simulink model "AE623_Burder_MakeupQuiz2_Problem2_LKF_EKF"  (R2016b)
settings: Solver=VariableStepAuto  StartTime=0.0  StopTime=10800  RelTol=1e-3
values from neighbouring files (symbols this model uses):
  T = 0.1    [AE623_Burder_MakeupQuiz2_Problem1.m]    (also in UKF.m = times)
undefined symbols (not defined in the file or in its folder): DiscIntNeverNeededParam
settings Model: Creator=burderd  LastModifiedBy=burderd

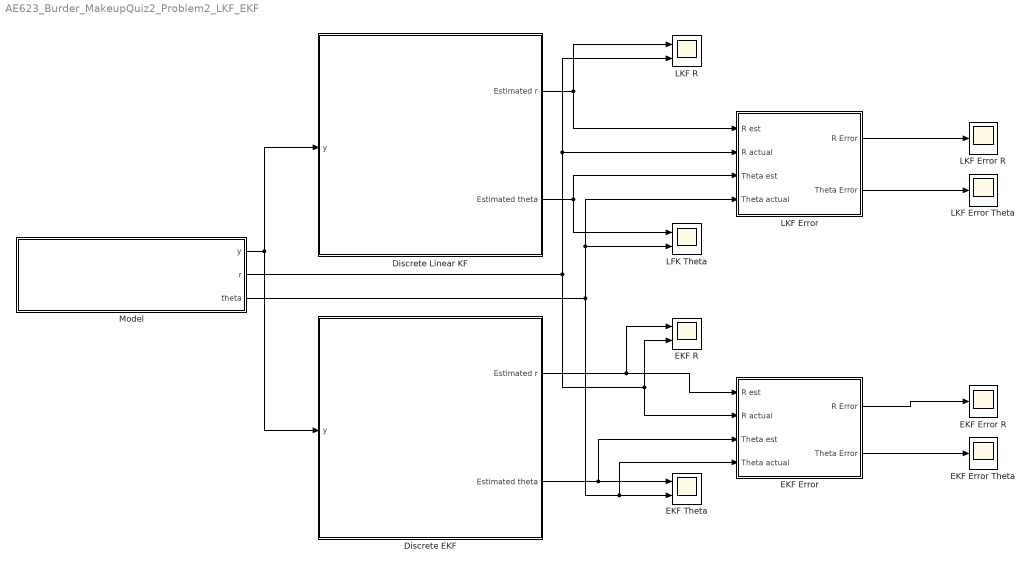
== system AE623_Burder_MakeupQuiz2_Problem2_LKF_EKF ==
  " EKF Error Theta" : Scope
  " EKF Theta" : Scope  NumInputPorts=2
  " LFK Theta" : Scope  NumInputPorts=2
  " LKF Error Theta" : Scope
  Discrete EKF : Subsystem  mask{Td=1, G=6.66742e-11, M=5.98e24, w0=0.011171034854823, r0=1.57e6}
  Discrete Linear KF : Subsystem  mask{Td=1, G=6.66742e-11, M=5.98e24, w0=0.011171034854823, r0=1.57e6}
  EKF Error : Subsystem
  EKF Error R : Scope
  EKF R : Scope  NumInputPorts=2
  LKF Error : Subsystem
  LKF Error R : Scope
  LKF R : Scope  NumInputPorts=2
  Model : Subsystem
  wires:
  Model/1(y) -> Discrete Linear KF/1(y), Discrete EKF/1(y)
  Discrete Linear KF/1(Estimated r) -> LKF R/1, LKF Error/1(R est)
  Discrete Linear KF/2(Estimated theta) -> LKF Error/3(Theta est), " LFK Theta"/1
  Model/2(r) -> EKF Error/2(R actual), EKF R/2, LKF R/2, LKF Error/2(R actual)
  Model/3(theta) -> " LFK Theta"/2, LKF Error/4(Theta actual), EKF Error/4(Theta actual), " EKF Theta"/2
  Discrete EKF/1(Estimated r) -> EKF Error/1(R est), EKF R/1
  Discrete EKF/2(Estimated theta) -> EKF Error/3(Theta est), " EKF Theta"/1
  LKF Error/1(R Error) -> LKF Error R/1
  LKF Error/2(Theta Error) -> " LKF Error Theta"/1
  EKF Error/1(R Error) -> EKF Error R/1
  EKF Error/2(Theta Error) -> " EKF Error Theta"/1

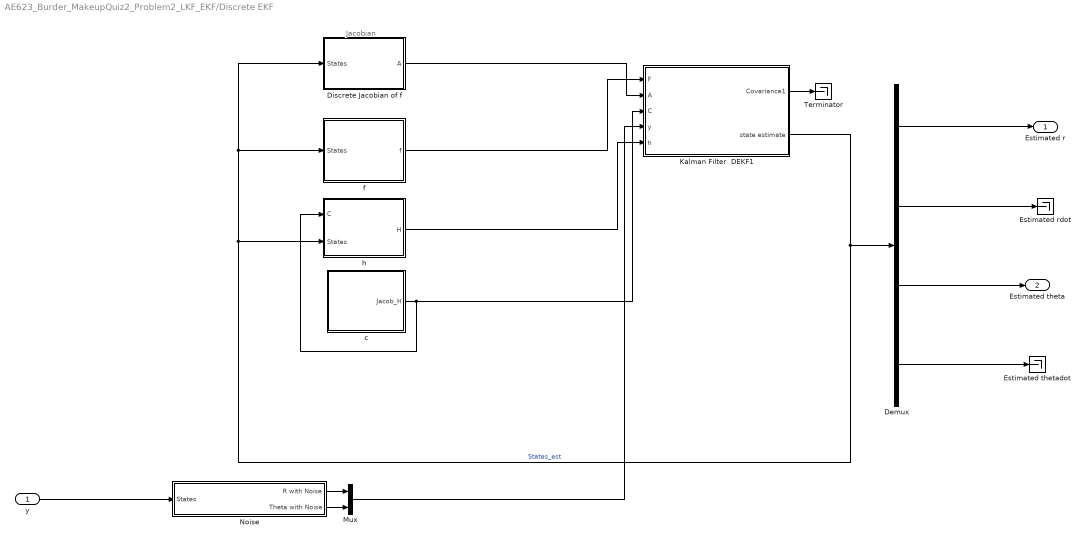
== system AE623_Burder_MakeupQuiz2_Problem2_LKF_EKF/Discrete EKF ==
  note: Jacobian
  y : Inport
  Demux : Demux
  Discrete Jacobian of f : Subsystem
  Estimated rdot : Terminator
  Estimated thetadot : Terminator
  Kalman Filter  DEKF1 : Subsystem
  Mux : Mux  Inputs=2
  Noise : Subsystem
  Terminator : Terminator
  c : Subsystem
  "f " : Subsystem
  h : Subsystem
  Estimated r : Outport
  Estimated theta : Outport  Port=2
  wires:
  Mux/1 -> Kalman Filter  DEKF1/4(y)
  y/1 -> Noise/1(States)
  Noise/2(Theta with Noise) -> Mux/2
  Noise/1(R with Noise) -> Mux/1
  h/1(H) -> Kalman Filter  DEKF1/5(h)
  Kalman Filter  DEKF1/2(state estimate) -> Demux/1, h/2(States), Discrete Jacobian of f/1(States), "f "/1(States)  "States_est"
  Kalman Filter  DEKF1/1(Covariance1) -> Terminator/1
  c/1(Jacob_H) -> h/1(C), Kalman Filter  DEKF1/3(C)
  "f "/1(f) -> Kalman Filter  DEKF1/1(F)
  Demux/1 -> Estimated r/1
  Demux/2 -> Estimated rdot/1
  Demux/3 -> Estimated theta/1
  Demux/4 -> Estimated thetadot/1
  Discrete Jacobian of f/1(A) -> Kalman Filter  DEKF1/2(A)

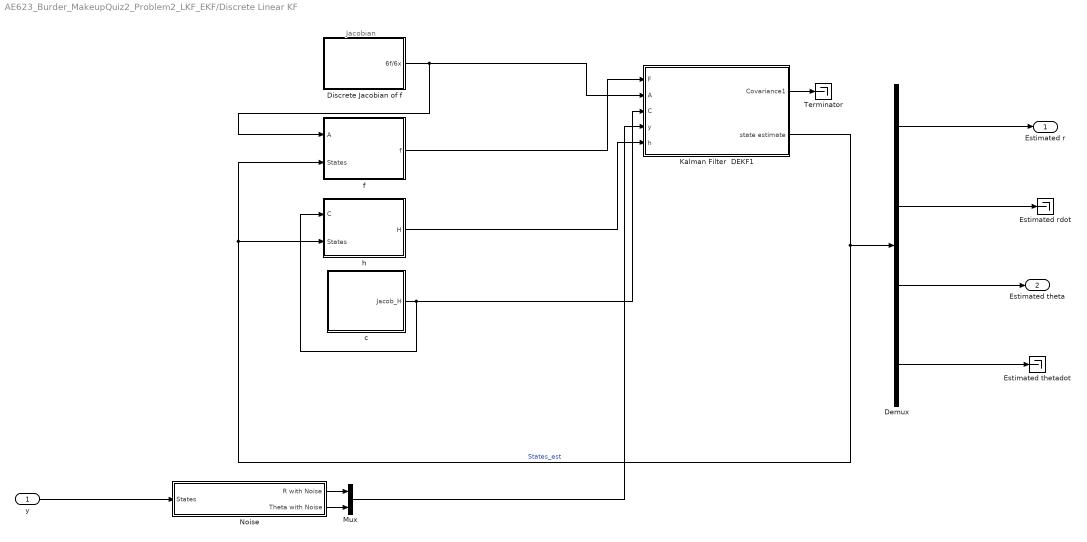
== system AE623_Burder_MakeupQuiz2_Problem2_LKF_EKF/Discrete Linear KF ==
  note: Jacobian
  y : Inport
  Demux : Demux
  Discrete Jacobian of f : Subsystem
  Estimated rdot : Terminator
  Estimated thetadot : Terminator
  Kalman Filter  DEKF1 : Subsystem
  Mux : Mux  Inputs=2
  Noise : Subsystem
  Terminator : Terminator
  c : Subsystem
  "f " : Subsystem
  h : Subsystem
  Estimated r : Outport
  Estimated theta : Outport  Port=2
  wires:
  Demux/4 -> Estimated thetadot/1
  Demux/3 -> Estimated theta/1
  Demux/2 -> Estimated rdot/1
  Demux/1 -> Estimated r/1
  Discrete Jacobian of f/1(6f/6x) -> Kalman Filter  DEKF1/2(A), "f "/1(A)
  "f "/1(f) -> Kalman Filter  DEKF1/1(F)
  c/1(Jacob_H) -> Kalman Filter  DEKF1/3(C), h/1(C)
  Kalman Filter  DEKF1/1(Covariance1) -> Terminator/1
  Kalman Filter  DEKF1/2(state estimate) -> "f "/2(States), h/2(States), Demux/1  "States_est"
  h/1(H) -> Kalman Filter  DEKF1/5(h)
  Noise/1(R with Noise) -> Mux/1
  Noise/2(Theta with Noise) -> Mux/2
  y/1 -> Noise/1(States)
  Mux/1 -> Kalman Filter  DEKF1/4(y)

== system AE623_Burder_MakeupQuiz2_Problem2_LKF_EKF/EKF Error ==
  R est : Inport
  R actual : Inport  Port=2
  Theta est : Inport  Port=3
  Theta actual : Inport  Port=4
  Sum2 : Sum  Inputs=|+-
  Sum3 : Sum  Inputs=|+-
  R Error : Outport
  Theta Error : Outport  Port=2
  wires:
  Theta est/1 -> Sum3/2
  R actual/1 -> Sum2/1
  R est/1 -> Sum2/2
  Theta actual/1 -> Sum3/1
  Sum2/1 -> R Error/1
  Sum3/1 -> Theta Error/1

== system AE623_Burder_MakeupQuiz2_Problem2_LKF_EKF/LKF Error ==
  R est : Inport
  R actual : Inport  Port=2
  Theta est : Inport  Port=3
  Theta actual : Inport  Port=4
  Sum2 : Sum  Inputs=|+-
  Sum3 : Sum  Inputs=|+-
  R Error : Outport
  Theta Error : Outport  Port=2
  wires:
  Theta est/1 -> Sum3/2
  R actual/1 -> Sum2/1
  R est/1 -> Sum2/2
  Theta actual/1 -> Sum3/1
  Sum2/1 -> R Error/1
  Sum3/1 -> Theta Error/1

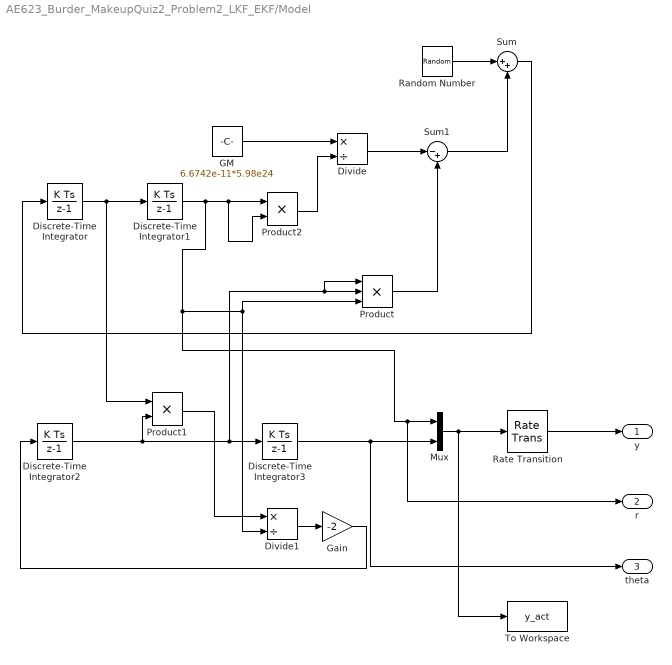
== system AE623_Burder_MakeupQuiz2_Problem2_LKF_EKF/Model ==
  Discrete-Time Integrator : DiscreteIntegrator  InitialConditionSetting=State (most efficient)  SampleTime=-1  ICPrevOutput=DiscIntNeverNeededParam  ICPrevScaledInput=DiscIntNeverNeededParam
  Discrete-Time Integrator1 : DiscreteIntegrator  InitialCondition=1.57e6  InitialConditionSetting=State (most efficient)  SampleTime=-1  ICPrevOutput=DiscIntNeverNeededParam  ICPrevScaledInput=DiscIntNeverNeededParam
  Discrete-Time Integrator2 : DiscreteIntegrator  InitialCondition=1.1*sqrt(6.6742e-11*5.98e24/(1.57e6)^3)  InitialConditionSetting=State (most efficient)  SampleTime=-1  ICPrevOutput=DiscIntNeverNeededParam  ICPrevScaledInput=DiscIntNeverNeededParam
  Discrete-Time Integrator3 : DiscreteIntegrator  InitialConditionSetting=State (most efficient)  SampleTime=-1  ICPrevOutput=DiscIntNeverNeededParam  ICPrevScaledInput=DiscIntNeverNeededParam
  Divide : Product  Inputs=*/
  Divide1 : Product  Inputs=*/
  GM : Constant  Value=6.6742e-11*5.98e24
  Gain : Gain  Gain=-2
  Mux : Mux  Inputs=2
  Product : Product  Inputs=3
  Product1 : Product
  Product2 : Product
  Random Number : RandomNumber  Variance=10e-6
  Rate Transition : RateTransition  X0=[1.57e6 0]  OutPortSampleTime=60
  Sum : Sum  Inputs=|++
  Sum1 : Sum  Inputs=|-+
  To Workspace : ToWorkspace  VariableName=y_act  SaveFormat=Timeseries  SampleTime=-1
  y : Outport
  r : Outport  Port=2
  theta : Outport  Port=3
  wires:
  Divide/1 -> Sum1/1
  Random Number/1 -> Sum/1
  GM/1 -> Divide/1
  Sum/1 -> Discrete-Time Integrator/1
  Sum1/1 -> Sum/2
  Discrete-Time Integrator/1 -> Product1/1, Discrete-Time Integrator1/1
  Discrete-Time Integrator3/1 -> theta/1, Mux/2
  Discrete-Time Integrator1/1 -> Product2/2, Product2/1, Divide1/2, Product/3, r/1, Mux/1
  Discrete-Time Integrator2/1 -> Product1/2, Product/1, Product/2, Discrete-Time Integrator3/1
  Mux/1 -> To Workspace/1, Rate Transition/1
  Product1/1 -> Divide1/1
  Divide1/1 -> Gain/1
  Product/1 -> Sum1/2
  Gain/1 -> Discrete-Time Integrator2/1
  Product2/1 -> Divide/2
  Rate Transition/1 -> y/1

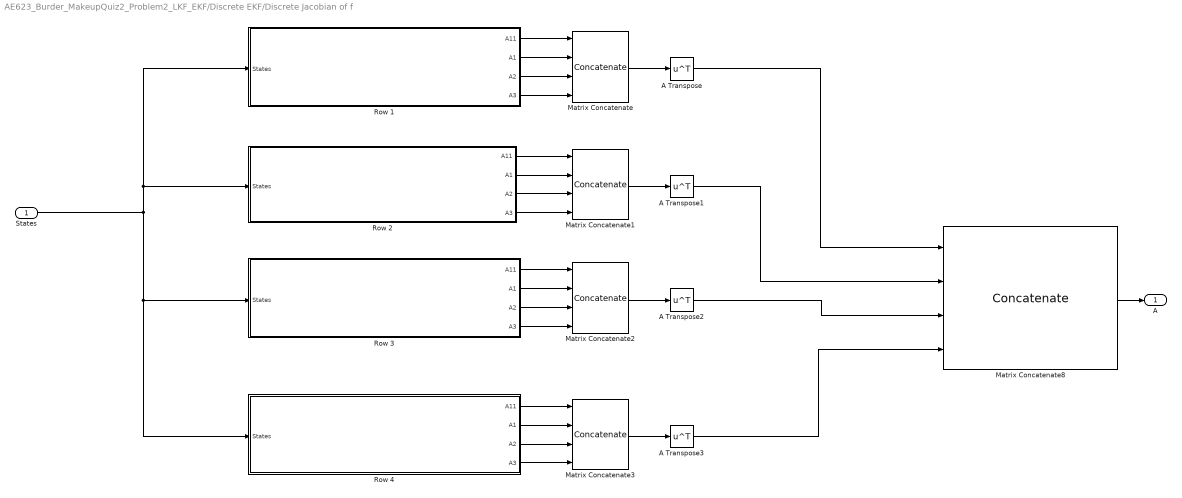
== system AE623_Burder_MakeupQuiz2_Problem2_LKF_EKF/Discrete EKF/Discrete Jacobian of f ==
  States : Inport
  A Transpose{,1..3} (4 alike) : Math  Operator=transpose  SaturateOnIntegerOverflow=on
  Matrix Concatenate{,1..3} (4 alike) : Concatenate  NumInputs=4  ConcatenateDimension=2
  Matrix Concatenate8 : Concatenate  NumInputs=4  Mode=Multidimensional array
  Row 1 : Subsystem
  Row 2 : Subsystem
  Row 3 : Subsystem
  Row 4 : Subsystem
  A : Outport
  wires:
  Matrix Concatenate8/1 -> A/1
  Row 1/1(A11) -> Matrix Concatenate/1
  Row 1/2(A1) -> Matrix Concatenate/2
  Row 1/3(A2) -> Matrix Concatenate/3
  Row 1/4(A3) -> Matrix Concatenate/4
  Matrix Concatenate/1 -> A Transpose/1
  A Transpose/1 -> Matrix Concatenate8/1
  Row 2/1(A11) -> Matrix Concatenate1/1
  Row 2/2(A1) -> Matrix Concatenate1/2
  Row 2/3(A2) -> Matrix Concatenate1/3
  Row 2/4(A3) -> Matrix Concatenate1/4
  Matrix Concatenate1/1 -> A Transpose1/1
  Row 3/1(A11) -> Matrix Concatenate2/1
  Row 3/2(A1) -> Matrix Concatenate2/2
  Row 3/3(A2) -> Matrix Concatenate2/3
  Row 3/4(A3) -> Matrix Concatenate2/4
  Matrix Concatenate2/1 -> A Transpose2/1
  Row 4/1(A11) -> Matrix Concatenate3/1
  Row 4/2(A1) -> Matrix Concatenate3/2
  Row 4/3(A2) -> Matrix Concatenate3/3
  Row 4/4(A3) -> Matrix Concatenate3/4
  Matrix Concatenate3/1 -> A Transpose3/1
  A Transpose1/1 -> Matrix Concatenate8/2
  A Transpose2/1 -> Matrix Concatenate8/3
  A Transpose3/1 -> Matrix Concatenate8/4
  States/1 -> Row 2/1(States), Row 1/1(States), Row 3/1(States), Row 4/1(States)

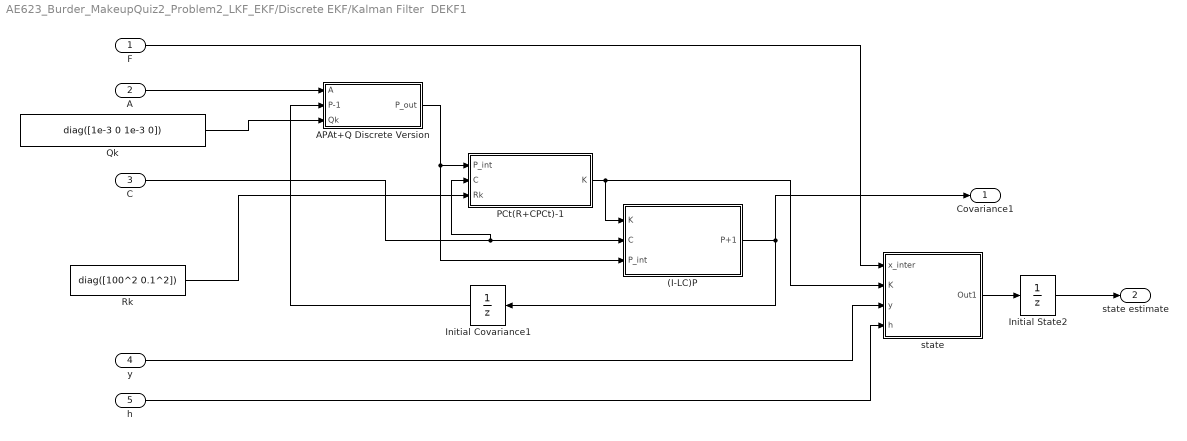
== system AE623_Burder_MakeupQuiz2_Problem2_LKF_EKF/Discrete EKF/Kalman Filter  DEKF1 ==
  F : Inport
  A : Inport  Port=2
  C : Inport  Port=3
  y : Inport  Port=4
  h : Inport  Port=5
  (I-LC)P : Subsystem
  APAt+Q Discrete Version : Subsystem
  Initial Covariance1 : UnitDelay  InitialCondition=zeros(4,4)  SampleTime=Td
  Initial State2 : UnitDelay  InitialCondition=[1.57e6 0 0 1.1*w0]  SampleTime=Td
  PCt(R+CPCt)-1 : Subsystem
  Qk : Constant  Value=diag([1e-3 0 1e-3 0])
  Rk : Constant  Value=diag([100^2 0.1^2])
  state : Subsystem
  Covariance1 : Outport
  state estimate : Outport  Port=2
  wires:
  F/1 -> state/1(x_inter)
  Initial State2/1 -> state estimate/1
  state/1(Out1) -> Initial State2/1
  Initial Covariance1/1 -> APAt+Q Discrete Version/2(P-1)
  PCt(R+CPCt)-1/1(K) -> (I-LC)P/1(K), state/2(K)
  (I-LC)P/1(P+1) -> Initial Covariance1/1, Covariance1/1
  Qk/1 -> APAt+Q Discrete Version/3(Qk)
  APAt+Q Discrete Version/1(P_out) -> (I-LC)P/3(P_int), PCt(R+CPCt)-1/1(P_int)
  A/1 -> APAt+Q Discrete Version/1(A)
  C/1 -> PCt(R+CPCt)-1/2(C), (I-LC)P/2(C)
  y/1 -> state/3(y)
  h/1 -> state/4(h)
  Rk/1 -> PCt(R+CPCt)-1/3(Rk)

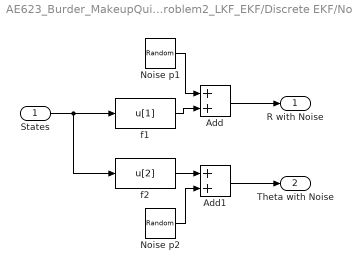
== system AE623_Burder_MakeupQuiz2_Problem2_LKF_EKF/Discrete EKF/Noise ==
  States : Inport
  Add : Sum
  Add1 : Sum
  Noise p1 : RandomNumber  Variance=100  Seed=565  SampleTime=T
  Noise p2 : RandomNumber  Variance=0.1  Seed=525  SampleTime=T
  f1 : Fcn  Expr=u[1]
  f2 : Fcn  Expr=u[2]
  R with Noise : Outport
  Theta with Noise : Outport  Port=2
  wires:
  f2/1 -> Add1/1
  Noise p2/1 -> Add1/2
  Add1/1 -> Theta with Noise/1
  States/1 -> f1/1, f2/1
  f1/1 -> Add/2
  Noise p1/1 -> Add/1
  Add/1 -> R with Noise/1

== system AE623_Burder_MakeupQuiz2_Problem2_LKF_EKF/Discrete EKF/c ==
  note: u[1] =p
      | u[2]=q
      | u[3]=r
      | u[4]=bank_est
      | u[5]=pitch_est
      | u[6]=heading_est
  Matrix Concatenate11 : Concatenate  Mode=Multidimensional array
  Row 1 : Subsystem
  Row 2 : Subsystem
  Jacob_H : Outport
  wires:
  Row 1/1(A11) -> Matrix Concatenate11/1
  Matrix Concatenate11/1 -> Jacob_H/1
  Row 2/1(A21) -> Matrix Concatenate11/2

== system AE623_Burder_MakeupQuiz2_Problem2_LKF_EKF/Discrete EKF/f  ==
  States : Inport
  Matrix Concatenate8 : Concatenate  NumInputs=4  Mode=Multidimensional array
  Row 1 : Subsystem
  Row 2 : Subsystem
  Row 3 : Subsystem
  Row 4 : Subsystem
  f : Outport
  wires:
  Matrix Concatenate8/1 -> f/1
  States/1 -> Row 2/1(States), Row 1/1(States), Row 3/1(States), Row 4/1(States)
  Row 1/1(A11) -> Matrix Concatenate8/1
  Row 2/1(A11) -> Matrix Concatenate8/2
  Row 3/1(A11) -> Matrix Concatenate8/3
  Row 4/1(A11) -> Matrix Concatenate8/4

== system AE623_Burder_MakeupQuiz2_Problem2_LKF_EKF/Discrete EKF/h ==
  C : Inport
  States : Inport  Port=2
  Matrix Multiply : Product  Multiplication=Matrix(*)
  H : Outport
  wires:
  Matrix Multiply/1 -> H/1
  C/1 -> Matrix Multiply/1
  States/1 -> Matrix Multiply/2

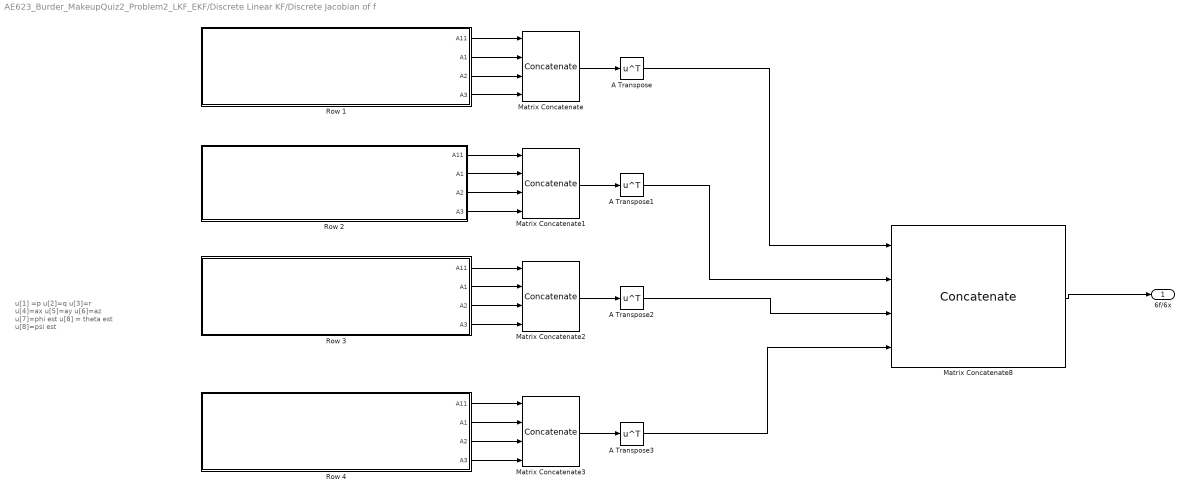
== system AE623_Burder_MakeupQuiz2_Problem2_LKF_EKF/Discrete Linear KF/Discrete Jacobian of f ==
  note: u[1] =p
      | u[2]=q
      | u[3]=r
      | u[4]=ax
      | u[5]=ay
      | u[6]=az
      | u[7]=phi est
      | u[8] = theta est
      | u[8]=psi est
  A Transpose{,1..3} (4 alike) : Math  Operator=transpose  SaturateOnIntegerOverflow=on
  Matrix Concatenate{,1..3} (4 alike) : Concatenate  NumInputs=4  ConcatenateDimension=2
  Matrix Concatenate8 : Concatenate  NumInputs=4  Mode=Multidimensional array
  Row 1 : Subsystem
  Row 2 : Subsystem
  Row 3 : Subsystem
  Row 4 : Subsystem
  6f/6x : Outport
  wires:
  A Transpose3/1 -> Matrix Concatenate8/4
  A Transpose2/1 -> Matrix Concatenate8/3
  A Transpose1/1 -> Matrix Concatenate8/2
  Matrix Concatenate3/1 -> A Transpose3/1
  Row 4/4(A3) -> Matrix Concatenate3/4
  Row 4/3(A2) -> Matrix Concatenate3/3
  Row 4/2(A1) -> Matrix Concatenate3/2
  Row 4/1(A11) -> Matrix Concatenate3/1
  Matrix Concatenate2/1 -> A Transpose2/1
  Row 3/4(A3) -> Matrix Concatenate2/4
  Row 3/3(A2) -> Matrix Concatenate2/3
  Row 3/2(A1) -> Matrix Concatenate2/2
  Row 3/1(A11) -> Matrix Concatenate2/1
  Matrix Concatenate1/1 -> A Transpose1/1
  Row 2/4(A3) -> Matrix Concatenate1/4
  Row 2/3(A2) -> Matrix Concatenate1/3
  Row 2/2(A1) -> Matrix Concatenate1/2
  Row 2/1(A11) -> Matrix Concatenate1/1
  A Transpose/1 -> Matrix Concatenate8/1
  Matrix Concatenate/1 -> A Transpose/1
  Row 1/4(A3) -> Matrix Concatenate/4
  Row 1/3(A2) -> Matrix Concatenate/3
  Row 1/2(A1) -> Matrix Concatenate/2
  Row 1/1(A11) -> Matrix Concatenate/1
  Matrix Concatenate8/1 -> 6f/6x/1

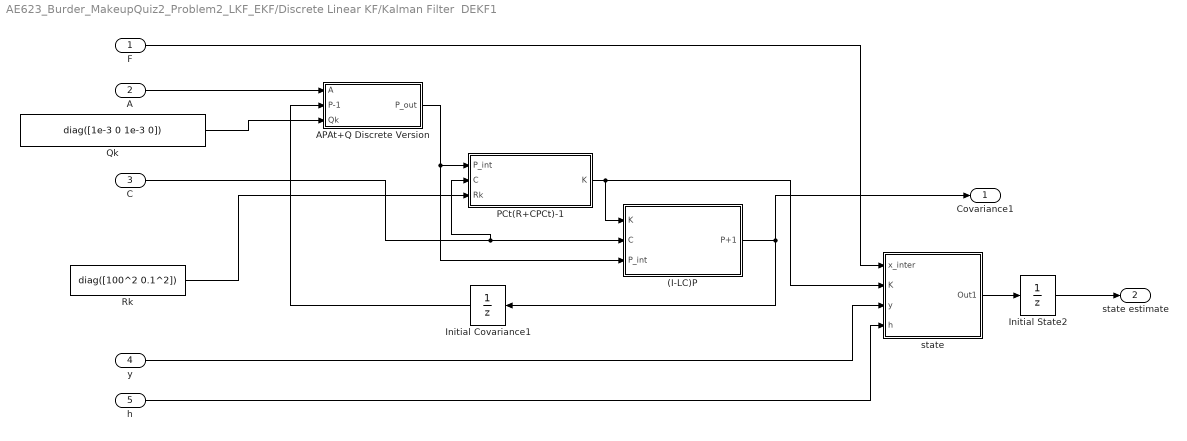
== system AE623_Burder_MakeupQuiz2_Problem2_LKF_EKF/Discrete Linear KF/Kalman Filter  DEKF1 ==
  F : Inport
  A : Inport  Port=2
  C : Inport  Port=3
  y : Inport  Port=4
  h : Inport  Port=5
  (I-LC)P : Subsystem
  APAt+Q Discrete Version : Subsystem
  Initial Covariance1 : UnitDelay  InitialCondition=zeros(4,4)  SampleTime=Td
  Initial State2 : UnitDelay  InitialCondition=[1.57e6 0 0 1.1*w0]  SampleTime=Td
  PCt(R+CPCt)-1 : Subsystem
  Qk : Constant  Value=diag([1e-3 0 1e-3 0])
  Rk : Constant  Value=diag([100^2 0.1^2])
  state : Subsystem
  Covariance1 : Outport
  state estimate : Outport  Port=2
  wires:
  Rk/1 -> PCt(R+CPCt)-1/3(Rk)
  h/1 -> state/4(h)
  y/1 -> state/3(y)
  C/1 -> (I-LC)P/2(C), PCt(R+CPCt)-1/2(C)
  A/1 -> APAt+Q Discrete Version/1(A)
  APAt+Q Discrete Version/1(P_out) -> PCt(R+CPCt)-1/1(P_int), (I-LC)P/3(P_int)
  Qk/1 -> APAt+Q Discrete Version/3(Qk)
  (I-LC)P/1(P+1) -> Covariance1/1, Initial Covariance1/1
  PCt(R+CPCt)-1/1(K) -> state/2(K), (I-LC)P/1(K)
  Initial Covariance1/1 -> APAt+Q Discrete Version/2(P-1)
  state/1(Out1) -> Initial State2/1
  Initial State2/1 -> state estimate/1
  F/1 -> state/1(x_inter)

== system AE623_Burder_MakeupQuiz2_Problem2_LKF_EKF/Discrete Linear KF/Noise ==
  States : Inport
  Add : Sum
  Add1 : Sum
  Noise p1 : RandomNumber  Variance=100  Seed=565  SampleTime=T
  Noise p2 : RandomNumber  Variance=0.1  Seed=525  SampleTime=T
  f1 : Fcn  Expr=u[1]
  f2 : Fcn  Expr=u[2]
  R with Noise : Outport
  Theta with Noise : Outport  Port=2
  wires:
  Add/1 -> R with Noise/1
  Noise p1/1 -> Add/1
  f1/1 -> Add/2
  States/1 -> f2/1, f1/1
  Add1/1 -> Theta with Noise/1
  Noise p2/1 -> Add1/2
  f2/1 -> Add1/1

== system AE623_Burder_MakeupQuiz2_Problem2_LKF_EKF/Discrete Linear KF/c ==
  note: u[1] =p
      | u[2]=q
      | u[3]=r
      | u[4]=bank_est
      | u[5]=pitch_est
      | u[6]=heading_est
  Matrix Concatenate11 : Concatenate  Mode=Multidimensional array
  Row 1 : Subsystem
  Row 2 : Subsystem
  Jacob_H : Outport
  wires:
  Row 2/1(A21) -> Matrix Concatenate11/2
  Matrix Concatenate11/1 -> Jacob_H/1
  Row 1/1(A11) -> Matrix Concatenate11/1

== system AE623_Burder_MakeupQuiz2_Problem2_LKF_EKF/Discrete Linear KF/f  ==
  A : Inport
  States : Inport  Port=2
  Matrix Multiply : Product  Multiplication=Matrix(*)
  f : Outport
  wires:
  States/1 -> Matrix Multiply/2
  A/1 -> Matrix Multiply/1
  Matrix Multiply/1 -> f/1

== system AE623_Burder_MakeupQuiz2_Problem2_LKF_EKF/Discrete Linear KF/h ==
  C : Inport
  States : Inport  Port=2
  Matrix Multiply : Product  Multiplication=Matrix(*)
  H : Outport
  wires:
  States/1 -> Matrix Multiply/2
  C/1 -> Matrix Multiply/1
  Matrix Multiply/1 -> H/1

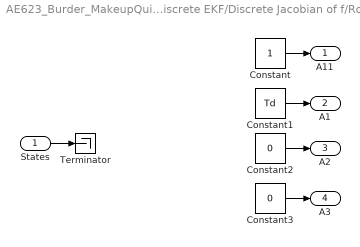
== system AE623_Burder_MakeupQuiz2_Problem2_LKF_EKF/Discrete EKF/Discrete Jacobian of f/Row 1 ==
  States : Inport
  Constant : Constant
  Constant1 : Constant  Value=Td
  Constant2 : Constant  Value=0
  Constant3 : Constant  Value=0
  Terminator : Terminator
  A11 : Outport
  A1 : Outport  Port=2
  A2 : Outport  Port=3
  A3 : Outport  Port=4
  wires:
  Constant/1 -> A11/1
  Constant1/1 -> A1/1
  Constant2/1 -> A2/1
  Constant3/1 -> A3/1
  States/1 -> Terminator/1

== system AE623_Burder_MakeupQuiz2_Problem2_LKF_EKF/Discrete EKF/Discrete Jacobian of f/Row 2 ==
  States : Inport
  Constant1 : Constant
  Constant2 : Constant  Value=0
  Fcn : Fcn  Expr=2*u(1)*u(4)*Td
  Fcn1 : Fcn  Expr=(2*G*M/((u(1))^3)+((u(4))^2))*Td
  A11 : Outport
  A1 : Outport  Port=2
  A2 : Outport  Port=3
  A3 : Outport  Port=4
  wires:
  Fcn/1 -> A3/1
  Constant2/1 -> A2/1
  Constant1/1 -> A1/1
  Fcn1/1 -> A11/1
  States/1 -> Fcn/1, Fcn1/1

== system AE623_Burder_MakeupQuiz2_Problem2_LKF_EKF/Discrete EKF/Discrete Jacobian of f/Row 3 ==
  States : Inport
  Constant : Constant  Value=0
  Constant1 : Constant  Value=0
  Constant2 : Constant
  Constant3 : Constant  Value=Td
  A11 : Outport
  A1 : Outport  Port=2
  A2 : Outport  Port=3
  A3 : Outport  Port=4
  wires:
  Constant/1 -> A11/1
  Constant1/1 -> A1/1
  Constant2/1 -> A2/1
  Constant3/1 -> A3/1

== system AE623_Burder_MakeupQuiz2_Problem2_LKF_EKF/Discrete EKF/Discrete Jacobian of f/Row 4 ==
  States : Inport
  Constant2 : Constant  Value=0
  Fcn : Fcn  Expr=1+2*u(2)*Td/u(1)
  Fcn1 : Fcn  Expr=-2*u(4)*Td/u(1)
  Fcn2 : Fcn  Expr=2*u(2)*u(4)*Td/(u(1)^2)
  A11 : Outport
  A1 : Outport  Port=2
  A2 : Outport  Port=3
  A3 : Outport  Port=4
  wires:
  Fcn/1 -> A3/1
  Constant2/1 -> A2/1
  Fcn1/1 -> A1/1
  Fcn2/1 -> A11/1
  States/1 -> Fcn2/1, Fcn1/1, Fcn/1

== system AE623_Burder_MakeupQuiz2_Problem2_LKF_EKF/Discrete EKF/Kalman Filter  DEKF1/(I-LC)P ==
  K : Inport
  C : Inport  Port=2
  P_int : Inport  Port=3
  I : Constant  Value=eye(4)
  Product1 : Product  Multiplication=Matrix(*)  SaturateOnIntegerOverflow=on  InputSameDT=on  OutDataTypeStr=Inherit: Same as first input
  Product2 : Product  Multiplication=Matrix(*)  SaturateOnIntegerOverflow=on  InputSameDT=on  OutDataTypeStr=Inherit: Same as first input
  Sum1 : Sum  Inputs=+-|
  P+1 : Outport
  wires:
  Product2/1 -> Sum1/2
  I/1 -> Sum1/1
  Sum1/1 -> Product1/1
  K/1 -> Product2/1
  C/1 -> Product2/2
  P_int/1 -> Product1/2
  Product1/1 -> P+1/1

== system AE623_Burder_MakeupQuiz2_Problem2_LKF_EKF/Discrete EKF/Kalman Filter  DEKF1/APAt+Q Discrete Version ==
  A : Inport
  P-1 : Inport  Port=2
  Qk : Inport  Port=3
  A Transpose : Math  Operator=transpose  SaturateOnIntegerOverflow=on
  Product1 : Product  Multiplication=Matrix(*)  SaturateOnIntegerOverflow=on  InputSameDT=on  OutDataTypeStr=Inherit: Same as first input
  Product2 : Product  Multiplication=Matrix(*)  SaturateOnIntegerOverflow=on  InputSameDT=on  OutDataTypeStr=Inherit: Same as first input
  Sum1 : Sum
  P_out : Outport
  wires:
  A/1 -> Product1/1, A Transpose/1
  P-1/1 -> Product1/2
  Product1/1 -> Product2/1
  A Transpose/1 -> Product2/2
  Sum1/1 -> P_out/1
  Qk/1 -> Sum1/2
  Product2/1 -> Sum1/1

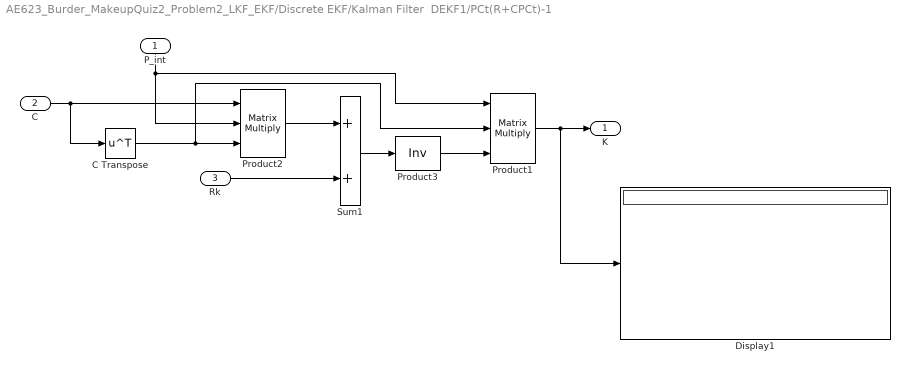
== system AE623_Burder_MakeupQuiz2_Problem2_LKF_EKF/Discrete EKF/Kalman Filter  DEKF1/PCt(R+CPCt)-1 ==
  P_int : Inport
  C : Inport  Port=2
  Rk : Inport  Port=3
  C Transpose : Math  Operator=transpose  SaturateOnIntegerOverflow=on
  Display1 : Display
  Product1 : Product  Inputs=3  Multiplication=Matrix(*)  SaturateOnIntegerOverflow=on  InputSameDT=on  OutDataTypeStr=Inherit: Same as first input
  Product2 : Product  Inputs=3  Multiplication=Matrix(*)  SaturateOnIntegerOverflow=on  InputSameDT=on  OutDataTypeStr=Inherit: Same as first input
  Product3 : Product  Inputs=/  Multiplication=Matrix(*)  SaturateOnIntegerOverflow=on  InputSameDT=on  OutDataTypeStr=Inherit: Same as first input
  Sum1 : Sum
  K : Outport
  wires:
  C/1 -> Product2/1, C Transpose/1
  C Transpose/1 -> Product2/3, Product1/2
  Product2/1 -> Sum1/1
  P_int/1 -> Product2/2, Product1/1
  Rk/1 -> Sum1/2
  Product3/1 -> Product1/3
  Sum1/1 -> Product3/1
  Product1/1 -> K/1, Display1/1

== system AE623_Burder_MakeupQuiz2_Problem2_LKF_EKF/Discrete EKF/Kalman Filter  DEKF1/state ==
  x_inter : Inport
  K : Inport  Port=2
  y : Inport  Port=3
  h : Inport  Port=4
  Product1 : Product  Multiplication=Matrix(*)  SaturateOnIntegerOverflow=on  InputSameDT=on  OutDataTypeStr=Inherit: Same as first input
  Sum1 : Sum  Inputs=|+-
  Sum2 : Sum  Inputs=++|
  Out1 : Outport
  wires:
  Sum1/1 -> Product1/2
  Product1/1 -> Sum2/2
  K/1 -> Product1/1
  x_inter/1 -> Sum2/1
  Sum2/1 -> Out1/1
  y/1 -> Sum1/1
  h/1 -> Sum1/2

== system AE623_Burder_MakeupQuiz2_Problem2_LKF_EKF/Discrete EKF/c/Row 1 ==
  A Transpose1 : Math  Operator=transpose  SaturateOnIntegerOverflow=on
  Constant : Constant  Value=[1 0 0 0]
  A11 : Outport
  wires:
  Constant/1 -> A Transpose1/1
  A Transpose1/1 -> A11/1

== system AE623_Burder_MakeupQuiz2_Problem2_LKF_EKF/Discrete EKF/c/Row 2 ==
  A Transpose1 : Math  Operator=transpose  SaturateOnIntegerOverflow=on
  Constant : Constant  Value=[0 0 1 0]
  A21 : Outport
  wires:
  Constant/1 -> A Transpose1/1
  A Transpose1/1 -> A21/1

== system AE623_Burder_MakeupQuiz2_Problem2_LKF_EKF/Discrete EKF/f /Row 1 ==
  States : Inport
  Fcn : Fcn  Expr=u[1]+(u[2]*Td)
  A11 : Outport
  wires:
  Fcn/1 -> A11/1
  States/1 -> Fcn/1

== system AE623_Burder_MakeupQuiz2_Problem2_LKF_EKF/Discrete EKF/f /Row 2 ==
  States : Inport
  Fcn1 : Fcn  Expr=u(2)+(u(1)*(u(4)^2)-(G*M/(u(1)^2)))*Td
  A11 : Outport
  wires:
  Fcn1/1 -> A11/1
  States/1 -> Fcn1/1

== system AE623_Burder_MakeupQuiz2_Problem2_LKF_EKF/Discrete EKF/f /Row 3 ==
  States : Inport
  Fcn : Fcn  Expr=u[3]+(u[4]*Td)
  A11 : Outport
  wires:
  Fcn/1 -> A11/1
  States/1 -> Fcn/1

== system AE623_Burder_MakeupQuiz2_Problem2_LKF_EKF/Discrete EKF/f /Row 4 ==
  States : Inport
  Fcn2 : Fcn  Expr=u[4]-((2*u[4]*u[2]/u[1])*Td)
  A11 : Outport
  wires:
  Fcn2/1 -> A11/1
  States/1 -> Fcn2/1

== system AE623_Burder_MakeupQuiz2_Problem2_LKF_EKF/Discrete Linear KF/Discrete Jacobian of f/Row 1 ==
  Constant : Constant
  Constant1 : Constant  Value=Td
  Constant2 : Constant  Value=0
  Constant3 : Constant  Value=0
  A11 : Outport
  A1 : Outport  Port=2
  A2 : Outport  Port=3
  A3 : Outport  Port=4
  wires:
  Constant3/1 -> A3/1
  Constant2/1 -> A2/1
  Constant1/1 -> A1/1
  Constant/1 -> A11/1

== system AE623_Burder_MakeupQuiz2_Problem2_LKF_EKF/Discrete Linear KF/Discrete Jacobian of f/Row 2 ==
  Constant : Constant  Value=3*G*M*Td/((1.57e6)^3)
  Constant1 : Constant
  Constant2 : Constant  Value=0
  Constant3 : Constant  Value=(sqrt(G*M/(1.57e6)))*(2*Td)
  A11 : Outport
  A1 : Outport  Port=2
  A2 : Outport  Port=3
  A3 : Outport  Port=4
  wires:
  Constant/1 -> A11/1
  Constant1/1 -> A1/1
  Constant2/1 -> A2/1
  Constant3/1 -> A3/1

== system AE623_Burder_MakeupQuiz2_Problem2_LKF_EKF/Discrete Linear KF/Discrete Jacobian of f/Row 3 ==
  Constant : Constant  Value=0
  Constant1 : Constant  Value=0
  Constant2 : Constant
  Constant3 : Constant  Value=Td
  A11 : Outport
  A1 : Outport  Port=2
  A2 : Outport  Port=3
  A3 : Outport  Port=4
  wires:
  Constant3/1 -> A3/1
  Constant2/1 -> A2/1
  Constant1/1 -> A1/1
  Constant/1 -> A11/1

== system AE623_Burder_MakeupQuiz2_Problem2_LKF_EKF/Discrete Linear KF/Discrete Jacobian of f/Row 4 ==
  Constant : Constant  Value=0
  Constant1 : Constant  Value=sqrt(G*M/(r0^5))*(-2*Td)
  Constant2 : Constant  Value=0
  Constant3 : Constant
  A11 : Outport
  A1 : Outport  Port=2
  A2 : Outport  Port=3
  A3 : Outport  Port=4
  wires:
  Constant/1 -> A11/1
  Constant1/1 -> A1/1
  Constant2/1 -> A2/1
  Constant3/1 -> A3/1

== system AE623_Burder_MakeupQuiz2_Problem2_LKF_EKF/Discrete Linear KF/Kalman Filter  DEKF1/(I-LC)P ==
  K : Inport
  C : Inport  Port=2
  P_int : Inport  Port=3
  I : Constant  Value=eye(4)
  Product1 : Product  Multiplication=Matrix(*)  SaturateOnIntegerOverflow=on  InputSameDT=on  OutDataTypeStr=Inherit: Same as first input
  Product2 : Product  Multiplication=Matrix(*)  SaturateOnIntegerOverflow=on  InputSameDT=on  OutDataTypeStr=Inherit: Same as first input
  Sum1 : Sum  Inputs=+-|
  P+1 : Outport
  wires:
  Product1/1 -> P+1/1
  P_int/1 -> Product1/2
  C/1 -> Product2/2
  K/1 -> Product2/1
  Sum1/1 -> Product1/1
  I/1 -> Sum1/1
  Product2/1 -> Sum1/2

== system AE623_Burder_MakeupQuiz2_Problem2_LKF_EKF/Discrete Linear KF/Kalman Filter  DEKF1/APAt+Q Discrete Version ==
  A : Inport
  P-1 : Inport  Port=2
  Qk : Inport  Port=3
  A Transpose : Math  Operator=transpose  SaturateOnIntegerOverflow=on
  Product1 : Product  Multiplication=Matrix(*)  SaturateOnIntegerOverflow=on  InputSameDT=on  OutDataTypeStr=Inherit: Same as first input
  Product2 : Product  Multiplication=Matrix(*)  SaturateOnIntegerOverflow=on  InputSameDT=on  OutDataTypeStr=Inherit: Same as first input
  Sum1 : Sum
  P_out : Outport
  wires:
  Product2/1 -> Sum1/1
  Qk/1 -> Sum1/2
  Sum1/1 -> P_out/1
  A Transpose/1 -> Product2/2
  Product1/1 -> Product2/1
  P-1/1 -> Product1/2
  A/1 -> A Transpose/1, Product1/1

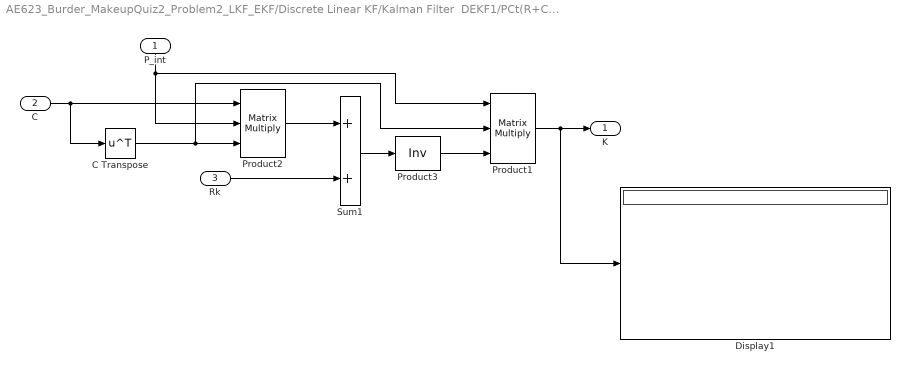
== system AE623_Burder_MakeupQuiz2_Problem2_LKF_EKF/Discrete Linear KF/Kalman Filter  DEKF1/PCt(R+CPCt)-1 ==
  P_int : Inport
  C : Inport  Port=2
  Rk : Inport  Port=3
  C Transpose : Math  Operator=transpose  SaturateOnIntegerOverflow=on
  Display1 : Display
  Product1 : Product  Inputs=3  Multiplication=Matrix(*)  SaturateOnIntegerOverflow=on  InputSameDT=on  OutDataTypeStr=Inherit: Same as first input
  Product2 : Product  Inputs=3  Multiplication=Matrix(*)  SaturateOnIntegerOverflow=on  InputSameDT=on  OutDataTypeStr=Inherit: Same as first input
  Product3 : Product  Inputs=/  Multiplication=Matrix(*)  SaturateOnIntegerOverflow=on  InputSameDT=on  OutDataTypeStr=Inherit: Same as first input
  Sum1 : Sum
  K : Outport
  wires:
  Product1/1 -> Display1/1, K/1
  Sum1/1 -> Product3/1
  Product3/1 -> Product1/3
  Rk/1 -> Sum1/2
  P_int/1 -> Product1/1, Product2/2
  Product2/1 -> Sum1/1
  C Transpose/1 -> Product1/2, Product2/3
  C/1 -> C Transpose/1, Product2/1

== system AE623_Burder_MakeupQuiz2_Problem2_LKF_EKF/Discrete Linear KF/Kalman Filter  DEKF1/state ==
  x_inter : Inport
  K : Inport  Port=2
  y : Inport  Port=3
  h : Inport  Port=4
  Product1 : Product  Multiplication=Matrix(*)  SaturateOnIntegerOverflow=on  InputSameDT=on  OutDataTypeStr=Inherit: Same as first input
  Sum1 : Sum  Inputs=|+-
  Sum2 : Sum  Inputs=++|
  Out1 : Outport
  wires:
  h/1 -> Sum1/2
  y/1 -> Sum1/1
  Sum2/1 -> Out1/1
  x_inter/1 -> Sum2/1
  K/1 -> Product1/1
  Product1/1 -> Sum2/2
  Sum1/1 -> Product1/2

== system AE623_Burder_MakeupQuiz2_Problem2_LKF_EKF/Discrete Linear KF/c/Row 1 ==
  A Transpose1 : Math  Operator=transpose  SaturateOnIntegerOverflow=on
  Constant : Constant  Value=[1 0 0 0]
  A11 : Outport
  wires:
  A Transpose1/1 -> A11/1
  Constant/1 -> A Transpose1/1

== system AE623_Burder_MakeupQuiz2_Problem2_LKF_EKF/Discrete Linear KF/c/Row 2 ==
  A Transpose1 : Math  Operator=transpose  SaturateOnIntegerOverflow=on
  Constant : Constant  Value=[0 0 1 0]
  A21 : Outport
  wires:
  A Transpose1/1 -> A21/1
  Constant/1 -> A Transpose1/1
